simulink model "aeropropmodel"  (Simulink 10.0)
settings: Solver=ode45  StartTime=0.0  StopTime=10.0  RelTol=1e-3  EnableMultiTasking=on
libraries: simulink3 x1, fdclib2 x1, fdclib3 x1
settings Model: Creator=bhisma  LastModifiedBy=bhisma  ExtModeTrigMode=oneshot  ExtModeArmWhenConnect=off
settings DataIOCC: SignalLoggingSaveFormat=ModelDataLogs
settings OptimizationCC: BlockReduction=off  BooleanDataType=off  LifeSpan=auto
settings DebuggingCC: SaveWithParameterizedLinksMsg=none  SignalResolutionControl=TryResolveAllWithWarning  MultiTaskDSMMsg=warning  MultiTaskCondExecSysMsg=none  SFUnexpectedBacktrackingDiag=error  SFNoUnconditionalDefaultTransitionDiag=error  SFExecutionAtInitializationDiag=warning  ArithmeticOperatorsInVariantConditions=error
settings HardwareCC: ProdBitPerPointer=64  ProdBitPerSizeT=64  ProdBitPerPtrDiffT=64  ProdLargestAtomicFloat=Float  ProdIntDivRoundTo=Zero  ProdEndianess=LittleEndian  ProdWordSize=64  ProdHWDeviceType=Intel->x86-64 (Windows64)  TargetUnknown=on
settings SFSimCC: SimUseLocalCustomCode=on  CustomCodeUndefinedFunction=FilterOut
settings RTWCC: RTWUseLocalCustomCode=on
settings CodeAppCC: StateflowObjectComments=off
settings GRTTargetCC: TargetLangStandard=C99 (ISO)
settings ConfigComp: CovMetricSettings=dwe  CovHtmlReporting=off  CovSaveCumulativeToWorkspaceVar=off  CovSaveSingleToWorkspaceVar=off

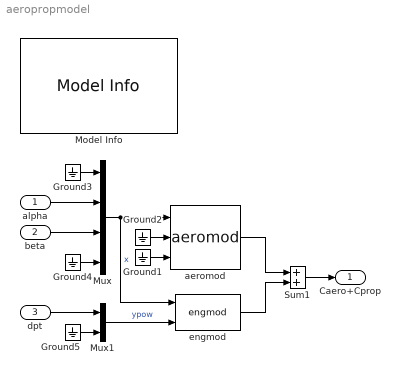
== system aeropropmodel ==
  alpha : Inport
  beta : Inport  Port=2
  dpt : Inport  Port=3
  Ground{1..5} (5 alike) : Ground
  Model Info : simulink3/Signals & Systems/Model Info  InitialBlockCM=none  BlockCM=none  Frame=on  DisplayStringWithTags=|  HorizontalTextAlignment=Center  LeftAlignmentValue=0.5  SourceBlockDiagram=aeropropmodel  TagMaxNumber=20
      | Test system to validate the 
      | aerodynamic and propulsive 
      | forces and moments models.
      | Used by PROPCOEFF.M.
      | 
      | M.O. Rauw, March 2004
      settings: SourceProductName=Simulink  SourceProductBaseCode=SL
  Mux : Mux  Inputs=[1 1 1 9]
  Mux1 : Mux  Inputs=2
  Sum1 : Sum  SaturateOnIntegerOverflow=on  InputSameDT=on  OutDataTypeStr=Inherit: Same as first input
  aeromod : fdclib2/aeromod
  engmod : fdclib3/engmod
  Caero+Cprop : Outport
  wires:
  aeromod/1 -> Sum1/1
  engmod/1 -> Sum1/2
  Sum1/1 -> Caero+Cprop/1
  Ground1/1 -> aeromod/3
  Ground2/1 -> aeromod/2
  Mux/1 -> aeromod/1, engmod/1  "x"
  alpha/1 -> Mux/2
  beta/1 -> Mux/3
  Ground3/1 -> Mux/1
  Ground4/1 -> Mux/4
  Mux1/1 -> engmod/2  "ypow"
  Ground5/1 -> Mux1/2
  dpt/1 -> Mux1/1
